simulink library "aero_librcs"  (Simulink 6.0)
settings: Solver=ode45  SolverMode=SingleTasking  StartTime=0.0  StopTime=10.0  RelTol=1e-3
values from neighbouring files (symbols this model uses):
  delt = clockt*160    (= 0.1)    [aero_dap3dofdata.m]
libraries: aero_libdap x3
settings Model: RequirementInfo=9  CovMetricSettings=d  Creator=The MathWorks Inc.  LastModifiedBy=batserve  ExtModeAutoUpdateStatusClock=off
settings OptimizationCC: BooleanDataType=off
settings DebuggingCC: AlgebraicLoopMsg=none  CheckExecutionContextPreStartOutputMsg=on  CheckExecutionContextRuntimeOutputMsg=on  SolverPrmCheckMsg=none
settings HardwareCC: TargetUnknown=on

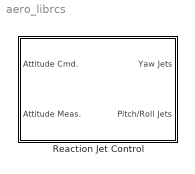
== system aero_librcs ==
  Reaction Jet Control : Subsystem  PropExecContextAcrossSSBoundary=on

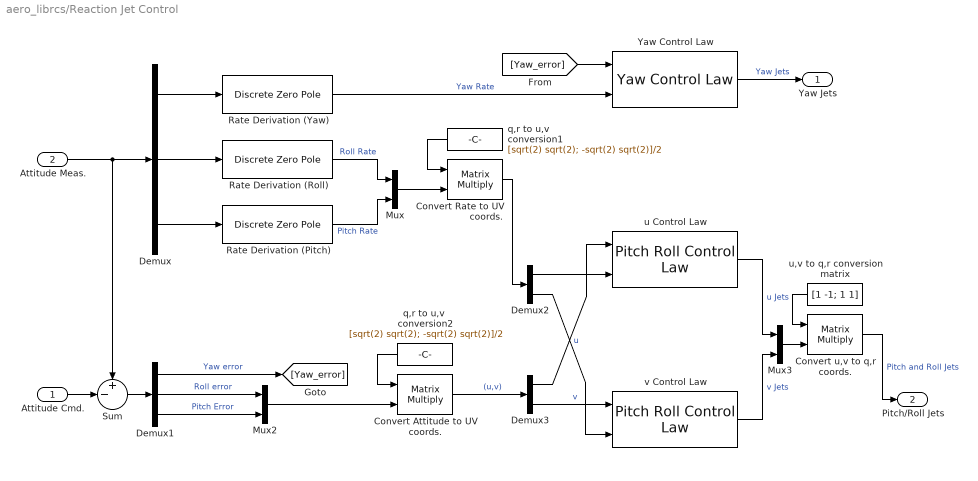
== system aero_librcs/Reaction Jet Control ==
  Attitude Cmd. : Inport  Port=1  LatchInput=off
  Attitude Meas. : Inport  Port=2  LatchInput=off
  Convert Attitude to UV coords. : Product  Multiplication=Matrix(*)  SaturateOnIntegerOverflow=on  RndMeth=Zero  InputSameDT=on
  Convert Rate to UV coords. : Product  Multiplication=Matrix(*)  SaturateOnIntegerOverflow=on  RndMeth=Zero  InputSameDT=on
  Convert u,v to q,r coords. : Product  Multiplication=Matrix(*)  SaturateOnIntegerOverflow=on  RndMeth=Zero  InputSameDT=on
  Demux : Demux  Outputs=3
  Demux1 : Demux  Outputs=3
  Demux2 : Demux  Outputs=2
  Demux3 : Demux  Outputs=2
  Mux : Mux  Inputs=2
  Mux2 : Mux  Inputs=2
  Mux3 : Mux  Inputs=2
  Rate Derivation (Pitch) : DiscreteZeroPole  Poles=[0]  Gain=1/delt  SampleTime=-1
  Rate Derivation (Roll) : DiscreteZeroPole  Poles=[0]  Gain=1/delt  SampleTime=-1
  Rate Derivation (Yaw) : DiscreteZeroPole  Poles=[0]  Gain=1/delt  SampleTime=-1
  Sum : Sum  Inputs=+-|  SaturateOnIntegerOverflow=on  InputSameDT=on
  Yaw Control Law : aero_libdap/Yaw Control Law  alph=alph1  alphs=alphs1  DB=DB  tmin=tmin  delt=delt
  q,r to u,v  conversion1 : Constant  Orientation=left  Value=[sqrt(2) sqrt(2); -sqrt(2) sqrt(2)]/2  VectorParams1D=off
  q,r to u,v  conversion2 : Constant  Orientation=left  Value=[sqrt(2) sqrt(2); -sqrt(2) sqrt(2)]/2  VectorParams1D=off
  u Control Law : aero_libdap/Pitch Roll Control Law  alph=alphu  alphs=alphsu  DB=DB  tmin=tmin  delt=delt
  u,v to q,r conversion matrix : Constant  Orientation=left  Value=[1 -1; 1 1]  VectorParams1D=off
  v Control Law : aero_libdap/Pitch Roll Control Law  alph=alphv  alphs=alphsv  DB=DB  tmin=tmin  delt=delt
  Yaw Jets : Outport  InitialOutput=0
  Pitch/Roll Jets : Outport  Port=2  InitialOutput=0
  wires:
  Demux3/1 -> u Control Law/1  "u"
  Convert u,v to q,r coords./1 -> Pitch/Roll Jets/1  "Pitch and Roll Jets"
  u,v to q,r conversion matrix/1 -> Convert u,v to q,r coords./1
  Mux3/1 -> Convert u,v to q,r coords./2
  Demux2/2 -> v Control Law/2
  Demux1/1 -> [Yaw_error]  "Yaw error"
  Demux2/1 -> u Control Law/2
  Demux3/2 -> v Control Law/1  "v"
  u Control Law/1 -> Mux3/1  "u Jets"
  v Control Law/1 -> Mux3/2  "v Jets"
  Attitude Cmd./1 -> Sum/2
  Mux2/1 -> Convert Attitude to UV coords./2
  Convert Attitude to UV coords./1 -> Demux3/1  "(u,v)"
  Convert Rate to UV coords./1 -> Demux2/1
  Demux1/3 -> Mux2/2  "Pitch Error"
  Demux1/2 -> Mux2/1  "Roll error"
  Sum/1 -> Demux1/1
  [Yaw_error] -> Yaw Control Law/1
  Yaw Control Law/1 -> Yaw Jets/1  "Yaw Jets"
  Rate Derivation (Yaw)/1 -> Yaw Control Law/2  "Yaw Rate"
  Attitude Meas./1 -> Sum/1, Demux/1
  Mux/1 -> Convert Rate to UV coords./2
  Demux/1 -> Rate Derivation (Yaw)/1
  Demux/3 -> Rate Derivation (Pitch)/1
  Demux/2 -> Rate Derivation (Roll)/1
  Rate Derivation (Roll)/1 -> Mux/1  "Roll Rate"
  Rate Derivation (Pitch)/1 -> Mux/2  "Pitch Rate"
  q,r to u,v  conversion1/1 -> Convert Rate to UV coords./1
  q,r to u,v  conversion2/1 -> Convert Attitude to UV coords./1
